simulink model "LabT1V2015b"  (R2015b)
settings: Solver=VariableStepAuto  SolverMode=SingleTasking  StartTime=0.0  StopTime=0.1  RelTol=1e-3
libraries: powerlib x38
settings Model: Creator=A.hey  LastModifiedBy=A.hey
settings DataIOCC: LimitDataPoints=off
settings DebuggingCC: AllowSymbolicDim=on  SFUnexpectedBacktrackingDiag=error  SFNoUnconditionalDefaultTransitionDiag=error
settings ModelReferenceCC: PropagateSignalLabelsOutOfModel=on
settings SFSimCC: SimUseLocalCustomCode=on
settings RTWCC: RTWUseLocalCustomCode=on
settings GRTTargetCC: TargetLangStandard=C99 (ISO)
settings ConfigComp: CovMetricSettings=dwe  CovHtmlReporting=off  CovSaveCumulativeToWorkspaceVar=off  CovSaveSingleToWorkspaceVar=off  CovModelRefEnable=Off  CovExternalEMLEnable=on
settings ConfigurationSet: Description=Simscape Multibody

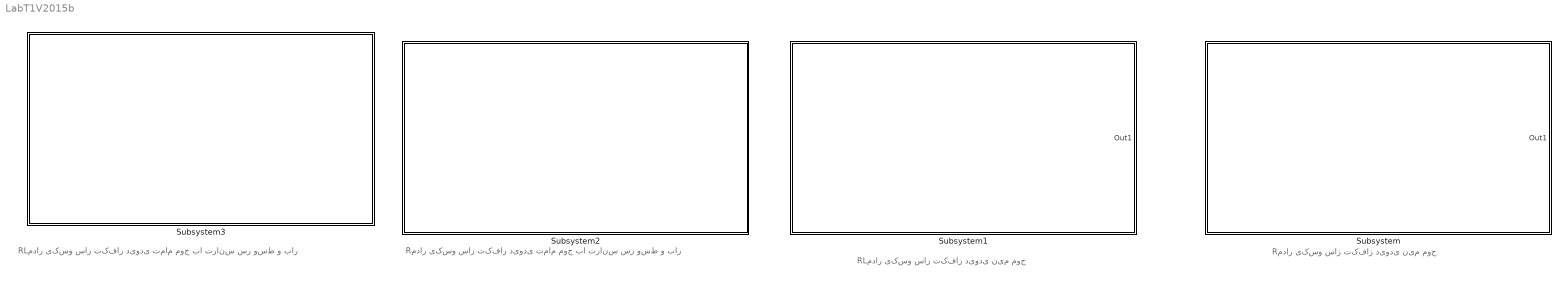
== system LabT1V2015b ==
  note: RLمدار یکسو ساز تکفاز دیودی نیم موج
  note: Rمدار یکسو ساز تکفاز دیودی نیم موج
  note: Rمدار یکسو ساز تکفاز دیودی تمام موج با ترانس سر وسط و بار
  note: RLمدار یکسو ساز تکفاز دیودی تمام موج با ترانس سر وسط و بار
  Subsystem : Subsystem
  Subsystem1 : Subsystem
  Subsystem2 : Subsystem
  Subsystem3 : Subsystem

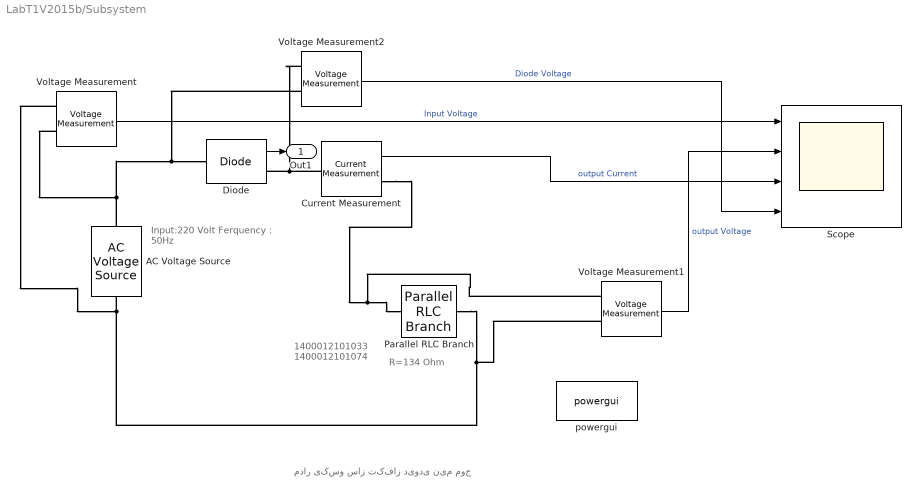
== system LabT1V2015b/Subsystem ==
  note: R=134 Ohm
  note: 1400012101033
      | 1400012101074
  note: Input:220 Volt
      | Ferquency : 50Hz
  note: مدار یکسو ساز تکفاز دیودی نیم موج
  AC Voltage Source : powerlib/Electrical Sources/AC Voltage Source  Amplitude=220  Phase=0  Frequency=50  SampleTime=0  Measurements=None  BusType=swing  Pref=10e3  Qref=0  Qmin=-inf  Qmax=+inf
  Current Measurement : powerlib/Measurements/Current Measurement  PhasorSimulation=off  OutputType=Complex  PSBequivalent=0
  Diode : powerlib/Power Electronics/Diode  Ron=0.001  Lon=0  Vf=0  IC=0  UseSnubber=0  Rs=500  Cs=250e-9  Measurements=on
  Parallel RLC Branch : powerlib/Elements/Parallel RLC Branch  LConnTagsString=a  RConnTagsString=__new0  BranchType=R  Resistance=134  Inductance=1e-3  SetiL0=off  InitialCurrent=0  Capacitance=1e-6  Setx0=off  InitialVoltage=0  Measurements=None
  Scope : Scope  NumInputPorts=4
  Voltage Measurement : powerlib/Measurements/Voltage Measurement  PhasorSimulation=off  OutputType=Complex  PSBequivalent=0
  Voltage Measurement1 : powerlib/Measurements/Voltage Measurement  PhasorSimulation=off  OutputType=Complex  PSBequivalent=0
  Voltage Measurement2 : powerlib/Measurements/Voltage Measurement  PhasorSimulation=off  OutputType=Complex  PSBequivalent=0
  powergui : powerlib/powergui  Priority=1  SimulationMode=Continuous  SampleTime=50e-6  frequency=60  Iterations=50  frequencyindice=50  Pbase=100e6  ErrMax=1e-4  UnitsV=kV  UnitsW=MW  buscounter=0  FunctionMessages=off  echomessages=off  EnableUseOfTLC=off  CurrentSourceSwitches=off  DisableSnubberDevices=off  DisableRonSwitches=off  DisableVfSwitches=off  DisplayEquations=off  SolverType=Tustin/Backward Euler (TBE)  Interpol=off  ExternalGateDelay=off  methode=off  Ts=100  x0status=blocks  SPID=on  SwTol=0  HookPort=off  RestoreLinks=warning  ResistiveCurrentMeasurement=off  Frange=[0:2:500]  Ylog=off  Xlog=on  ShowGrid=off  save=off  variable=ZData  structure=0  ZoomFFT=off  StartTime=0.0  cycles=1  DisplayStyle=1  fundamental=60  FreqAxis=off  MaxFrequency=1000  frequencyindicesteady=1  RmsSteady=1  display=off
  Out1 : Outport
  wires:
  Voltage Measurement/1 -> Scope/1  "Input Voltage"
  Current Measurement/1 -> Scope/3  "output Current"
  Diode/1 -> Out1/1
  Voltage Measurement2/1 -> Scope/4  "Diode Voltage"
  Voltage Measurement1/1 -> Scope/2  "output Voltage"
  connections:
  Current Measurement/LConn1 -- Voltage Measurement2/LConn2 -- Diode/RConn1
  Parallel RLC Branch/RConn1 -- Voltage Measurement1/LConn2 -- Voltage Measurement/LConn2 -- AC Voltage Source/LConn1
  Current Measurement/RConn1 -- Voltage Measurement1/LConn1 -- Parallel RLC Branch/LConn1
  AC Voltage Source/RConn1 -- Voltage Measurement/LConn1 -- Voltage Measurement2/LConn1 -- Diode/LConn1

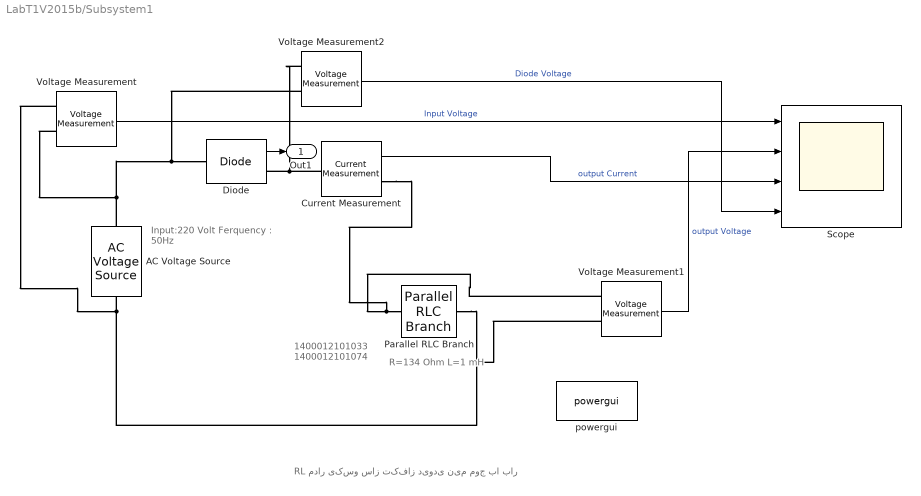
== system LabT1V2015b/Subsystem1 ==
  note: R=134 Ohm
      | L=1 mH
  note: 1400012101033
      | 1400012101074
  note: Input:220 Volt
      | Ferquency : 50Hz
  note: RL مدار یکسو ساز تکفاز دیودی نیم موج با بار
  AC Voltage Source : powerlib/Electrical Sources/AC Voltage Source  Amplitude=220  Phase=0  Frequency=50  SampleTime=0  Measurements=None  BusType=swing  Pref=10e3  Qref=0  Qmin=-inf  Qmax=+inf
  Current Measurement : powerlib/Measurements/Current Measurement  PhasorSimulation=off  OutputType=Complex  PSBequivalent=0
  Diode : powerlib/Power Electronics/Diode  Ron=0.001  Lon=0  Vf=0  IC=0  UseSnubber=0  Rs=500  Cs=250e-9  Measurements=on
  Parallel RLC Branch : powerlib/Elements/Parallel RLC Branch  LConnTagsString=a  RConnTagsString=__new0  BranchType=RL  Resistance=134  Inductance=1  SetiL0=off  InitialCurrent=0  Capacitance=1e-6  Setx0=off  InitialVoltage=0  Measurements=None
  Scope : Scope  NumInputPorts=4
  Voltage Measurement : powerlib/Measurements/Voltage Measurement  PhasorSimulation=off  OutputType=Complex  PSBequivalent=0
  Voltage Measurement1 : powerlib/Measurements/Voltage Measurement  PhasorSimulation=off  OutputType=Complex  PSBequivalent=0
  Voltage Measurement2 : powerlib/Measurements/Voltage Measurement  PhasorSimulation=off  OutputType=Complex  PSBequivalent=0
  powergui : powerlib/powergui  Priority=1  SimulationMode=Continuous  SampleTime=50e-6  frequency=60  Iterations=50  frequencyindice=50  Pbase=100e6  ErrMax=1e-4  UnitsV=kV  UnitsW=MW  buscounter=0  FunctionMessages=off  echomessages=off  EnableUseOfTLC=off  CurrentSourceSwitches=off  DisableSnubberDevices=off  DisableRonSwitches=off  DisableVfSwitches=off  DisplayEquations=off  SolverType=Tustin/Backward Euler (TBE)  Interpol=off  ExternalGateDelay=off  methode=off  Ts=100  x0status=blocks  SPID=on  SwTol=0  HookPort=off  RestoreLinks=warning  ResistiveCurrentMeasurement=off  Frange=[0:2:500]  Ylog=off  Xlog=on  ShowGrid=off  save=off  variable=ZData  structure=0  ZoomFFT=off  StartTime=0.0  cycles=1  DisplayStyle=1  fundamental=60  FreqAxis=off  MaxFrequency=1000  frequencyindicesteady=1  RmsSteady=1  display=off
  Out1 : Outport
  wires:
  Voltage Measurement/1 -> Scope/1  "Input Voltage"
  Current Measurement/1 -> Scope/3  "output Current"
  Diode/1 -> Out1/1
  Voltage Measurement2/1 -> Scope/4  "Diode Voltage"
  Voltage Measurement1/1 -> Scope/2  "output Voltage"
  connections:
  Current Measurement/LConn1 -- Diode/RConn1 -- Voltage Measurement2/LConn2
  Parallel RLC Branch/RConn1 -- Voltage Measurement/LConn2 -- AC Voltage Source/LConn1 -- Voltage Measurement1/LConn2
  Parallel RLC Branch/LConn1 -- Current Measurement/RConn1 -- Voltage Measurement1/LConn1
  Voltage Measurement/LConn1 -- AC Voltage Source/RConn1 -- Diode/LConn1 -- Voltage Measurement2/LConn1

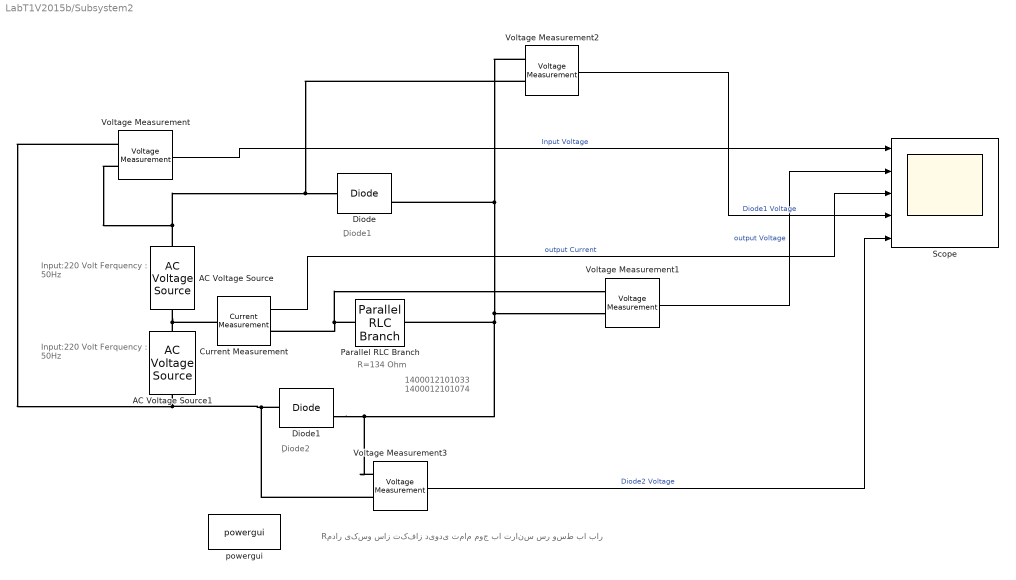
== system LabT1V2015b/Subsystem2 ==
  note: R=134 Ohm
  note: 1400012101033
      | 1400012101074
  note: Input:220 Volt
      | Ferquency : 50Hz
  note: Rمدار یکسو ساز تکفاز دیودی تمام موج با ترانس سر وسط با بار
  note: Input:220 Volt
      | Ferquency : 50Hz
  note: ِDiode2
  note: ِDiode1
  AC Voltage Source : powerlib/Electrical Sources/AC Voltage Source  Amplitude=220  Phase=0  Frequency=50  SampleTime=0  Measurements=None  BusType=swing  Pref=10e3  Qref=0  Qmin=-inf  Qmax=+inf
  AC Voltage Source1 : powerlib/Electrical Sources/AC Voltage Source  Amplitude=220  Phase=0  Frequency=50  SampleTime=0  Measurements=None  BusType=swing  Pref=10e3  Qref=0  Qmin=-inf  Qmax=+inf
  Current Measurement : powerlib/Measurements/Current Measurement  PhasorSimulation=off  OutputType=Complex  PSBequivalent=0
  Diode : powerlib/Power Electronics/Diode  Ron=0.001  Lon=0  Vf=0  IC=0  UseSnubber=0  Rs=500  Cs=250e-9  Measurements=on
  Diode1 : powerlib/Power Electronics/Diode  Ron=0.001  Lon=0  Vf=0  IC=0  UseSnubber=0  Rs=500  Cs=250e-9  Measurements=on
  Parallel RLC Branch : powerlib/Elements/Parallel RLC Branch  LConnTagsString=a  RConnTagsString=__new0  BranchType=R  Resistance=134  Inductance=1  SetiL0=off  InitialCurrent=0  Capacitance=1e-6  Setx0=off  InitialVoltage=0  Measurements=None
  Scope : Scope  NumInputPorts=5
  Voltage Measurement{,1..3} (4 alike) : powerlib/Measurements/Voltage Measurement  PhasorSimulation=off  OutputType=Complex  PSBequivalent=0
  powergui : powerlib/powergui  Priority=1  SimulationMode=Continuous  SampleTime=50e-6  frequency=60  Iterations=50  frequencyindice=50  Pbase=100e6  ErrMax=1e-4  UnitsV=kV  UnitsW=MW  buscounter=0  FunctionMessages=off  echomessages=off  EnableUseOfTLC=off  CurrentSourceSwitches=off  DisableSnubberDevices=off  DisableRonSwitches=off  DisableVfSwitches=off  DisplayEquations=off  SolverType=Tustin/Backward Euler (TBE)  Interpol=off  ExternalGateDelay=off  methode=off  Ts=100  x0status=blocks  SPID=on  SwTol=0  HookPort=off  RestoreLinks=warning  ResistiveCurrentMeasurement=off  Frange=[0:2:500]  Ylog=off  Xlog=on  ShowGrid=off  save=off  variable=ZData  structure=0  ZoomFFT=off  StartTime=0.0  cycles=1  DisplayStyle=1  fundamental=60  FreqAxis=off  MaxFrequency=1000  frequencyindicesteady=1  RmsSteady=1  display=off
  wires:
  Voltage Measurement/1 -> Scope/1  "Input Voltage"
  Current Measurement/1 -> Scope/3  "output Current"
  Voltage Measurement2/1 -> Scope/4  "Diode1 Voltage"
  Voltage Measurement1/1 -> Scope/2  "output Voltage"
  Voltage Measurement3/1 -> Scope/5  "Diode2 Voltage"
  connections:
  Parallel RLC Branch/LConn1 -- Voltage Measurement1/LConn2 -- Current Measurement/RConn1
  Voltage Measurement/LConn1 -- AC Voltage Source/RConn1 -- Voltage Measurement2/LConn1 -- Diode/LConn1
  Voltage Measurement/LConn2 -- Voltage Measurement3/LConn1 -- Diode1/LConn1 -- AC Voltage Source1/LConn1
  Voltage Measurement2/LConn2 -- Voltage Measurement1/LConn1 -- Voltage Measurement3/LConn2 -- Diode1/RConn1 -- Parallel RLC Branch/RConn1 -- Diode/RConn1
  AC Voltage Source1/RConn1 -- Current Measurement/LConn1 -- AC Voltage Source/LConn1

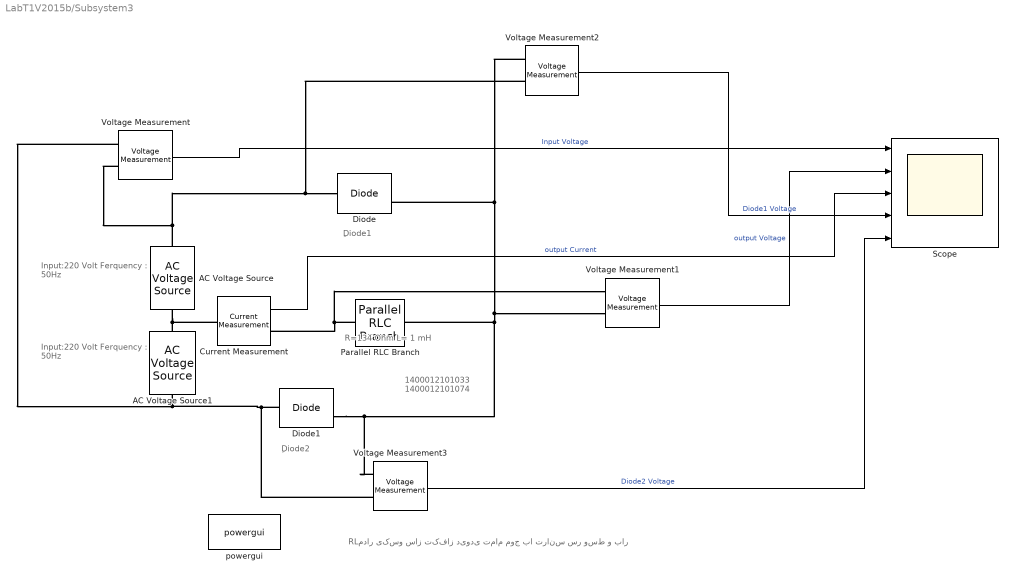
== system LabT1V2015b/Subsystem3 ==
  note: R=134 Ohm
      | L= 1 mH
  note: 1400012101033
      | 1400012101074
  note: Input:220 Volt
      | Ferquency : 50Hz
  note: Input:220 Volt
      | Ferquency : 50Hz
  note: ِDiode2
  note: ِDiode1
  note: RLمدار یکسو ساز تکفاز دیودی تمام موج با ترانس سر وسط و بار
  AC Voltage Source : powerlib/Electrical Sources/AC Voltage Source  Amplitude=220  Phase=0  Frequency=50  SampleTime=0  Measurements=None  BusType=swing  Pref=10e3  Qref=0  Qmin=-inf  Qmax=+inf
  AC Voltage Source1 : powerlib/Electrical Sources/AC Voltage Source  Amplitude=220  Phase=0  Frequency=50  SampleTime=0  Measurements=None  BusType=swing  Pref=10e3  Qref=0  Qmin=-inf  Qmax=+inf
  Current Measurement : powerlib/Measurements/Current Measurement  PhasorSimulation=off  OutputType=Complex  PSBequivalent=0
  Diode : powerlib/Power Electronics/Diode  Ron=0.001  Lon=0  Vf=0  IC=0  UseSnubber=0  Rs=500  Cs=250e-9  Measurements=on
  Diode1 : powerlib/Power Electronics/Diode  Ron=0.001  Lon=0  Vf=0  IC=0  UseSnubber=0  Rs=500  Cs=250e-9  Measurements=on
  Parallel RLC Branch : powerlib/Elements/Parallel RLC Branch  LConnTagsString=a  RConnTagsString=__new0  BranchType=RL  Resistance=134  Inductance=1e-3  SetiL0=off  InitialCurrent=0  Capacitance=1e-6  Setx0=off  InitialVoltage=0  Measurements=None
  Scope : Scope  NumInputPorts=5
  Voltage Measurement{,1..3} (4 alike) : powerlib/Measurements/Voltage Measurement  PhasorSimulation=off  OutputType=Complex  PSBequivalent=0
  powergui : powerlib/powergui  Priority=1  SimulationMode=Continuous  SampleTime=50e-6  frequency=60  Iterations=50  frequencyindice=50  Pbase=100e6  ErrMax=1e-4  UnitsV=kV  UnitsW=MW  buscounter=0  FunctionMessages=off  echomessages=off  EnableUseOfTLC=off  CurrentSourceSwitches=off  DisableSnubberDevices=off  DisableRonSwitches=off  DisableVfSwitches=off  DisplayEquations=off  SolverType=Tustin/Backward Euler (TBE)  Interpol=off  ExternalGateDelay=off  methode=off  Ts=100  x0status=blocks  SPID=on  SwTol=0  HookPort=off  RestoreLinks=warning  ResistiveCurrentMeasurement=off  Frange=[0:2:500]  Ylog=off  Xlog=on  ShowGrid=off  save=off  variable=ZData  structure=0  ZoomFFT=off  StartTime=0.0  cycles=1  DisplayStyle=1  fundamental=60  FreqAxis=off  MaxFrequency=1000  frequencyindicesteady=1  RmsSteady=1  display=off
  wires:
  Voltage Measurement/1 -> Scope/1  "Input Voltage"
  Current Measurement/1 -> Scope/3  "output Current"
  Voltage Measurement2/1 -> Scope/4  "Diode1 Voltage"
  Voltage Measurement1/1 -> Scope/2  "output Voltage"
  Voltage Measurement3/1 -> Scope/5  "Diode2 Voltage"
  connections:
  Current Measurement/RConn1 -- Parallel RLC Branch/LConn1 -- Voltage Measurement1/LConn2
  Voltage Measurement/LConn1 -- AC Voltage Source/RConn1 -- Diode/LConn1 -- Voltage Measurement2/LConn1
  AC Voltage Source1/LConn1 -- Voltage Measurement/LConn2 -- Diode1/LConn1 -- Voltage Measurement3/LConn1
  Voltage Measurement2/LConn2 -- Diode/RConn1 -- Voltage Measurement3/LConn2 -- Diode1/RConn1 -- Parallel RLC Branch/RConn1 -- Voltage Measurement1/LConn1
  AC Voltage Source1/RConn1 -- Current Measurement/LConn1 -- AC Voltage Source/LConn1
